simulink model "robot_model"  (R2025a)
settings: Solver=ode45  StartTime=0  StopTime=17  FixedStep=0.001  MaxStep=0.001  RelTol=1e-3
values from neighbouring files (symbols this model uses):
  K = table_of_controller_parameters(i).K    [plot_mesh_K.m]    (also in run_lqr_controller_optimization.m = table_of_controller_parameters(idx).K; run_the_robot_model.m = table_of_controller_parameters(idx).K)
  model_parameters = define_model_parameters()    [run_startup.m]    (also in startup.m)
libraries: simulink x6
settings Model: Creator=brzan  LastModifiedBy=brzan

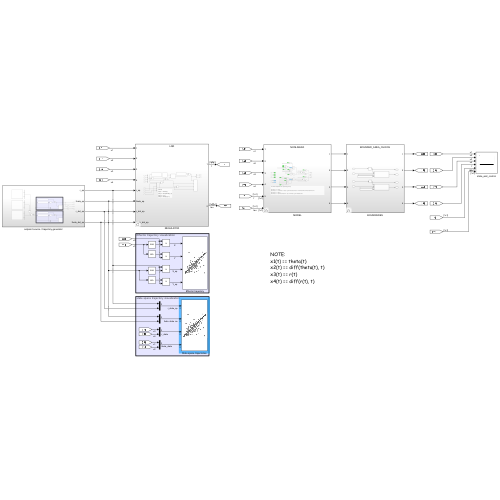
[thumbnail: Simulink's stored preview of the top-level diagram]
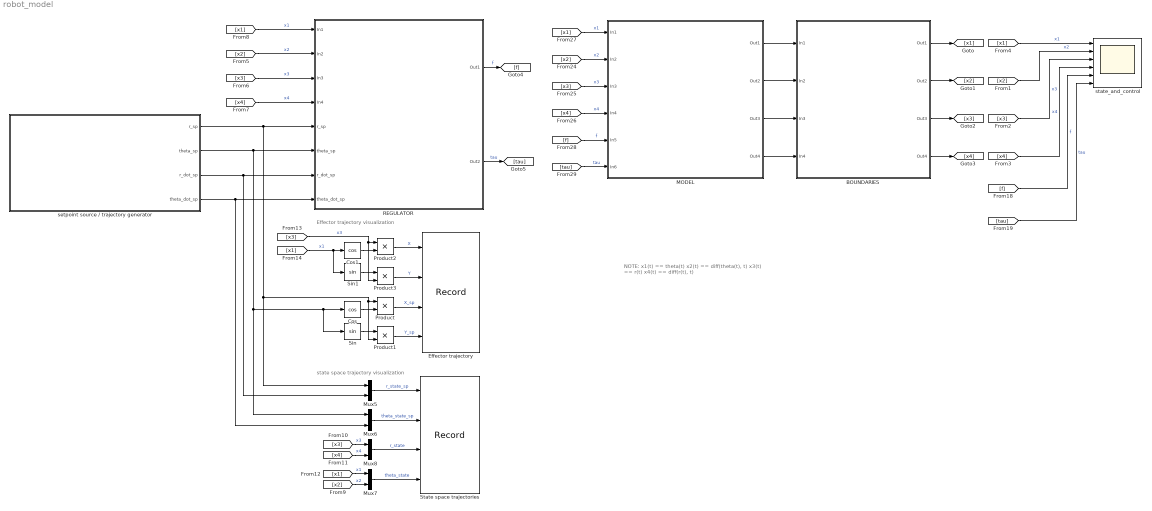
== system robot_model ==
  note: Effector trajectory visualization
  note: NOTE:
      | x1(t) == theta(t)
      | x2(t) == diff(theta(t), t)
      | x3(t) == r(t)
      | x4(t) == diff(r(t), t)
  note: state space trajectory visualization
  BOUNDARIES : Subsystem  Variant=on
  Cos : Trigonometry  Operator=cos
  Cos1 : Trigonometry  Operator=cos
  Effector trajectory : Record  NumPorts=4.0  FileSettingsInternal="{\"entries\":[{\"content\":{\"excelSettings\":{\"content\":{},\"type\":\"Streamout.ExcelSettings\"},\"parquetSettings\":{\"content\":{},\"type\":\"Streamout.ParquetSettings\"}},\"type\":\"Streamout.FileSettingStorage\",\"uuid\":\"\"}],\"packageUris\":[\"http:\\/\\/schema.mathworks.com\\/mf0\\/streamout_blocks\\/R2020a\"],\"version\":\"1.0\"}"  FrameSettings=[0, 0, 0, 0]  Layout=[1 2]  SignalsInternal="{\"entries\":[{\"content\":{\"signals\":[{\"content\":{\"blockPath\":[],\"dimensions\":[1],\"domain\":\"\",\"lineColor\":\"#0072bd\",\"plots\":[ 1 ],\"port\":1,\"sid\":[\"\"],\"signalID\":1,\"signalName\":\"X\"},\"type\":\"RecordBlkView.Signal\",\"uuid\":\"\"},{\"content\":{\"blockPath\":[],\"dimensions\":[1],\"domain\":\"\",\"lineColor\":\"#139fff\",\"plots\":[ 1 ],\"port\":2,\"sid\":[\"\"],\"signalID\":2,\"signalName\":\"Y\"},\"type\":\"RecordBlkView.Signal\",\"uuid\":\"\"},{\"content\":{\"blockPath\":[],\"dimensions\":[1],\"domain\":\"\",\"lineColor\":\"#d95319\",\"lineWidth\":2,\"plots\":[ 1 ],\"port\":3,\"sid\":[\"\"],\"signalID\":3,\"signalName\":\"X_sp\"},\"type\":\"RecordBlkView.Signal\",\"uuid\":\"\"},{\"content\":{\"blockPath\":[],\"dimensions\":[1],\"domain\":\"\",\"lineColor\":\"#ff6929\",\"lineWidth\":2,\"plots\":[ 1 ],\"port\":4,\"sid\":[\"\"],\"signalID\":4,\"signalName\":\"Y_sp\"},\"type\":\"RecordBlkView.Signal\",\"uuid\":\"\"}]},\"type\":\"RecordBlkView.InputSignals\",\"uuid\":\"\"}],\"packageUris\":[\"http:\\/\\/schema.mathworks.com\\/mf0\\/streamout_blocks\\/R2020a\"],\"version\":\"1.0\"}"  VisualizationBindings="{\"xyplotplugin\":{\"info\":[{\"series\":[{\"bindingParametersList\":[{\"parameter\":\"X-Axis\",\"signalID\":1,\"signalName\":\"X\"},{\"parameter\":\"Y-Axis\",\"signalID\":2,\"signalName\":\"Y\"}],\"seriesID\":0},{\"bindingParametersList\":[{\"parameter\":\"X-Axis\",\"signalID\":3,\"signalName\":\"X_sp\"},{\"parameter\":\"Y-Axis\",\"signalID\":4,\"signalName\":\"Y_sp\"}],\"seriesID\":1}],\"subplotID\":1}]}}"  CompatibilityTag=XY
  MODEL : Subsystem  Variant=on
  Mux{5..8} (4 alike) : Mux  Inputs=2
  Product{,1..3} (4 alike) : Product
  REGULATOR : Subsystem  Variant=on
  Sin : Trigonometry
  Sin1 : Trigonometry
  State space trajectories : Record  NumPorts=4.0  FileSettingsInternal="{\"entries\":[{\"content\":{\"excelSettings\":{\"content\":{},\"type\":\"Streamout.ExcelSettings\"},\"parquetSettings\":{\"content\":{},\"type\":\"Streamout.ParquetSettings\"}},\"type\":\"Streamout.FileSettingStorage\",\"uuid\":\"\"}],\"packageUris\":[\"http:\\/\\/schema.mathworks.com\\/mf0\\/streamout_blocks\\/R2020a\"],\"version\":\"1.0\"}"  FrameSettings=[0, 0, 0, 0]  Layout=[2 2]  SignalsInternal="{\"entries\":[{\"content\":{\"signals\":[{\"content\":{\"blockPath\":[],\"dimensions\":[2],\"domain\":\"\",\"hasChildren\":true,\"lineColor\":\"#ff6929\",\"lineWidth\":2,\"port\":1,\"sid\":[\"\"],\"signalID\":1,\"signalName\":\"r_state_sp\"},\"type\":\"RecordBlkView.Signal\",\"uuid\":\"\"},{\"content\":{\"blockPath\":[],\"channel\":[1],\"dimensions\":[2],\"domain\":\"\",\"lineColor\":\"#ff13a6\",\"lineWidth\":2,\"parentID\":1,\"plots\":[ 1, 9 ],\"port\":1,\"sid\":[\"\"],\"signalID\":2,\"signalName\":\"r_state_sp\"},\"type\":\"RecordBlkView.Signal\",\"uuid\":\"\"},{\"content\":{\"blockPath\":[],\"dimensions\":[2],\"domain\":\"\",\"hasChildren\":true,\"lineColor\":\"#64d413\",\"lineWidth\":2,\"port\":2,\"sid\":[\"\"],\"signalID\":3,\"signalName\":\"theta_state_sp\"},\"type\":\"RecordBlkView.Signal\",\"uuid\":\"\"},{\"content\":{\"blockPath\":[],\"channel\":[1],\"dimensions\":[2],\"domain\":\"\",\"lineColor\":\"#22b573\",\"lineWidth\":2,\"parentID\":3,\"plots\":[ 2, 10, 23 ],\"port\":2,\"sid\":[\"\"],\"signalID\":4,\"signalName\":\"theta_state_sp\"},\"type\":\"RecordBlkView.Signal\",\"uuid\":\"\"},{\"content\":{\"blockPath\":[],\"dimensions\":[2],\"domain\":\"\",\"hasChildren\":true,\"lineColor\":\"#fe330a\",\"lineWidth\":2,\"port\":3,\"sid\":[\"\"],\"signalID\":5,\"signalName\":\"r_state\"},\"type\":\"RecordBlkView.Signal\",\"uuid\":\"\"},{\"content\":{\"blockPath\":[],\"channel\":[1],\"dimensions\":[2],\"domain\":\"\",\"lineColor\":\"#d95319\",\"lineWidth\":2,\"parentID\":5,\"plots\":[ 1, 3, 5, 9, 25 ],\"port\":3,\"sid\":[\"\"],\"signalID\":6,\"signalName\":\"r_state\"},\"type\":\"RecordBlkView.Signal\",\"uuid\":\"\"},{\"content\":{\"blockPath\":[],\"dimensions\":[2],\"domain\":\"\",\"hasChildren\":true,\"lineColor\":\"#0072bd\",\"lineWidth\":2,\"port\":4,\"sid\":[\"\"],\"signalID\":7,\"signalName\":\"theta_state\"},\"type\":\"RecordBlkView.Signal\",\"uuid\":\"\"},{\"content\":{\"blockPath\":[],\"channel\":[1],\"dimensions\":[2],\"domain\":\"\",\"lineColor\":\"#7e2f8e\",\"lineWidth\":2,\"parentID\":7,\"plots\":[ 2, 10, 26, 51 ],\"port\":4,\"sid\":[\"\"],\"signalID\":8,\"signalName\":\"theta_state\"},\"type\":\"RecordBlkView.Signal\",\"uuid\":\"\"},{\"content\":{\"blockPath\":[],\"channel\":[2],\"dimensions\":[2],\"domain\":\"\",\"lineColor\":\"#fe330a\",\"lineWidth\":2,\"parentID\":1,\"plots\":[ 1, 9, 15, 48 ],\"port\":1,\"sid\":[\"\"],\"signalID\":9,\"signalName\":\"r_state_sp\"},\"type\":\"RecordBlkView.Signal\",\"uuid\":\"\"},{\"content\":{\"blockPath\":[],\"channel\":[2],\"dimensions\":[2],\"domain\":\"\",\"lineColor\":\"#22b573\",\"lineWidth\":2,\"parentID\":3,\"plots\":[ 2, 10, 58, 59 ],\"port\":2,\"sid\":[\"\"],\"signalID\":10,\"signalName\":\"theta_state_sp\"},\"type\":\"RecordBlkView.Signal\",\"uuid\":\"\"},{\"content\":{\"blockPath\":[],\"channel\":[2],\"dimensions\":[2],\"domain\":\"\",\"lineColor\":\"#0072bd\",\"lineWidth\":2,\"parentID\":5,\"plots\":[ 1, 9, 41 ],\"port\":3,\"sid\":[\"\"],\"signalID\":11,\"signalName\":\"r_state\"},\"type\":\"RecordBlkView.Signal\",\"uuid\":\"\"},{\"content\":{\"blockPath\":[],\"channel\":[2],\"dimensions\":[2],\"domain\":\"\",\"lineColor\":\"#d95319\",\"lineWidth\":2,\"parentID\":7,\"plots\":[ 2, 10, 45 ],\"port\":4,\"sid\":[\"\"],\"signalID\":12,\"signalName\":\"theta_state\"},\"type\":\"RecordBlkView.Signal\",\"uuid\":\"\"}]},\"type\":\"RecordBlkView.InputSignals\",\"uuid\":\"\"}],\"packageUris\":[\"http:\\/\\/schema.mathworks.com\\/mf0\\/streamout_blocks\\/R2020a\"],\"version\":\"1.0\"}"  VisualizationBindings="{\"sparklinesplugin\":{\"info\":[{\"bindingParametersList\":[],\"subplotID\":9},{\"bindingParametersList\":[],\"subplotID\":10}]},\"xyplotplugin\":{\"info\":[{\"series\":[{\"bindingParametersList\":[{\"parameter\":\"X-Axis\",\"signalID\":2,\"signalName\":\"r_state_sp(1)\"},{\"parameter\":\"Y-Axis\",\"signalID\":9,\"signalName\":\"r_state_sp(2)\"}],\"seriesID\":0},{\"bindingParametersList\":[{\"parameter\":\"X-Axis\",\"signalID\":6,\"signalName\":\"r_state(1)\"},{\"parameter\":\"Y-Axis\",\"signalID\":11,\"signalName\":\"r_state(2)\"}],\"seriesID\":1}],\"subplotID\":1},{\"series\":[{\"bindingParametersList\":[{\"parameter\":\"X-Axis\",\"signalID\":4,\"signalName\":\"theta_state_sp(1)\"},{\"parameter\":\"Y-Axis\",\"signalID\":10,\"signalName\":\"theta_state_sp(2)\"}],\"seriesID\":2},{\"bindingParametersList\":[{\"parameter\":\"X-Axis\",\"signalID\":8,\"signalName\":\"theta_state(1)\"},{\"parameter\":\"Y-Axis\",\"signalID\":12,\"signalName\":\"theta_state(2)\"}],\"seriesID\":3}],\"subplotID\":2}]}}"  CompatibilityTag=XY
  setpoint source / trajectory generator : Subsystem
  state_and_control : Scope  NumInputPorts=6
      settings: ActiveDisplayYMinimum=2.4867230453181195  ActiveDisplayYMaximum=2.7484021064636068  DataLoggingVariableName=state_and_control
  wires:
  [x4] -> state_and_control/4  "x4"
  [x3] -> state_and_control/3  "x3"
  [x2] -> state_and_control/2  "x2"
  [x1] -> state_and_control/1  "x1"
  [f] -> state_and_control/5  "f"
  [tau] -> state_and_control/6  "tau"
  MODEL/1(Out1) -> BOUNDARIES/1(In1)
  MODEL/2(Out2) -> BOUNDARIES/2(In2)
  MODEL/3(Out3) -> BOUNDARIES/3(In3)
  MODEL/4(Out4) -> BOUNDARIES/4(In4)
  BOUNDARIES/1(Out1) -> [x1]
  BOUNDARIES/2(Out2) -> [x2]
  BOUNDARIES/3(Out3) -> [x3]
  BOUNDARIES/4(Out4) -> [x4]
  [x4] -> MODEL/4(In4)  "x4"
  [x3] -> MODEL/3(In3)  "x3"
  [x2] -> MODEL/2(In2)  "x2"
  [x1] -> MODEL/1(In1)  "x1"
  [f] -> MODEL/5(In5)  "f"
  [tau] -> MODEL/6(In6)  "tau"
  REGULATOR/2(Out2) -> [tau]  "tau"
  REGULATOR/1(Out1) -> [f]  "f"
  [x1] -> REGULATOR/1(In1)  "x1"
  [x2] -> REGULATOR/2(In2)  "x2"
  [x3] -> REGULATOR/3(In3)  "x3"
  [x4] -> REGULATOR/4(In4)  "x4"
  Cos/1 -> Product/2
  Sin/1 -> Product1/1
  Product/1 -> Effector trajectory/3  "X_sp"
  Product1/1 -> Effector trajectory/4  "Y_sp"
  Mux5/1 -> State space trajectories/1  "r_state_sp"
  Mux6/1 -> State space trajectories/2  "theta_state_sp"
  Mux8/1 -> State space trajectories/3  "r_state"
  Mux7/1 -> State space trajectories/4  "theta_state"
  [x1] -> Mux7/1  "x1"
  [x2] -> Mux7/2  "x2"
  [x4] -> Mux8/2  "x4"
  [x3] -> Mux8/1  "x3"
  [x1] -> Sin1/1, Cos1/1  "x1"
  [x3] -> Product3/2, Product2/1  "x3"
  Sin1/1 -> Product3/1
  Cos1/1 -> Product2/2
  Product3/1 -> Effector trajectory/2  "Y"
  Product2/1 -> Effector trajectory/1  "X"
  setpoint source / trajectory generator/2(theta_sp) -> Mux6/1, Cos/1, Sin/1, REGULATOR/6(theta_sp)
  setpoint source / trajectory generator/1(r_sp) -> Mux5/1, Product1/2, Product/1, REGULATOR/5(r_sp)
  setpoint source / trajectory generator/3(r_dot_sp) -> Mux5/2, REGULATOR/7(r_dot_sp)
  setpoint source / trajectory generator/4(theta_dot_sp) -> Mux6/2, REGULATOR/8(theta_dot_sp)

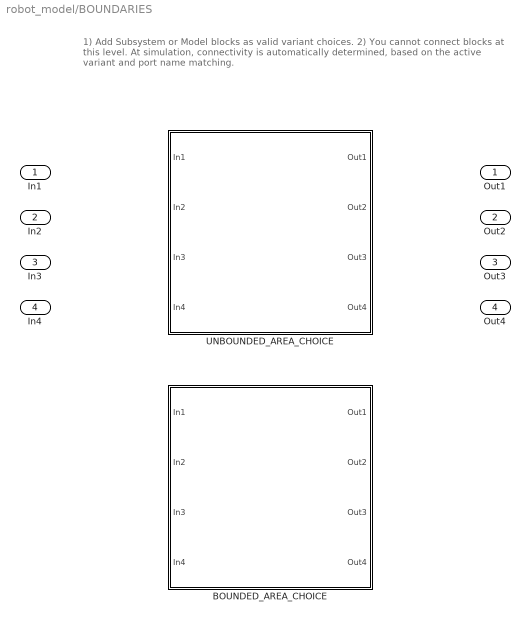
== system robot_model/BOUNDARIES ==
  note: 1) Add Subsystem or Model blocks as valid variant choices.
      | 2) You cannot connect blocks at this level. At simulation, connectivity is automatically
      | determined, based on the active variant and port name matching.
  In1 : Inport
  In2 : Inport  Port=2
  In3 : Inport  Port=3
  In4 : Inport  Port=4
  BOUNDED_AREA_CHOICE : Subsystem  VariantControl="BOUNDARY_CHOICE == \"BOUNDED\""
  UNBOUNDED_AREA_CHOICE : Subsystem  VariantControl="BOUNDARY_CHOICE == \"UNBOUNDED\""
  Out1 : Outport
  Out2 : Outport  Port=2
  Out3 : Outport  Port=3
  Out4 : Outport  Port=4

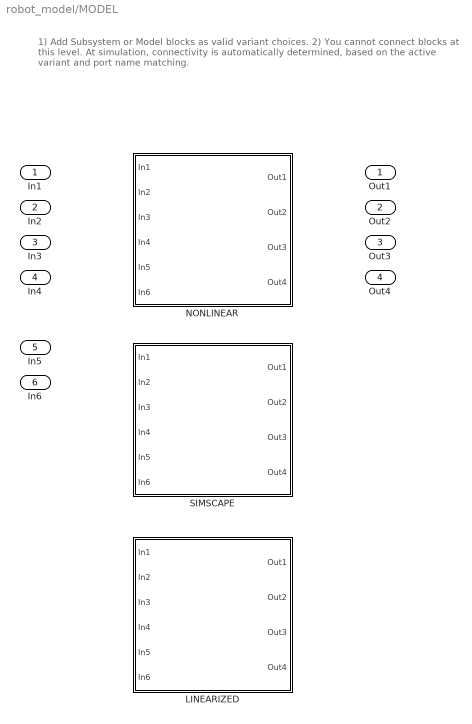
== system robot_model/MODEL ==
  note: 1) Add Subsystem or Model blocks as valid variant choices.
      | 2) You cannot connect blocks at this level. At simulation, connectivity is automatically
      | determined, based on the active variant and port name matching.
  In1 : Inport
  In2 : Inport  Port=2
  In3 : Inport  Port=3
  In4 : Inport  Port=4
  In5 : Inport  Port=5
  In6 : Inport  Port=6
  LINEARIZED : Subsystem  VariantControl="MODEL_CHOICE == \"LINEARIZED\""
  NONLINEAR : Subsystem  VariantControl="MODEL_CHOICE == \"NONLINEAR\""
  SIMSCAPE : Subsystem  VariantControl="MODEL_CHOICE == \"SIMSCAPE\""
  Out1 : Outport
  Out2 : Outport  Port=2
  Out3 : Outport  Port=3
  Out4 : Outport  Port=4

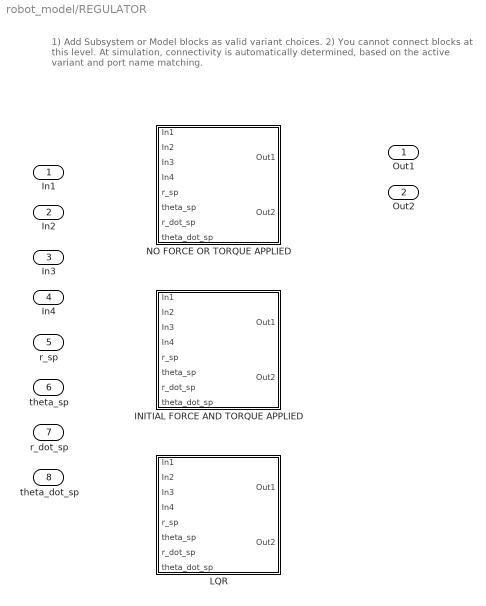
== system robot_model/REGULATOR ==
  note: 1) Add Subsystem or Model blocks as valid variant choices.
      | 2) You cannot connect blocks at this level. At simulation, connectivity is automatically
      | determined, based on the active variant and port name matching.
  In1 : Inport
  In2 : Inport  Port=2
  In3 : Inport  Port=3
  In4 : Inport  Port=4
  r_sp : Inport  Port=5
  theta_sp : Inport  Port=6
  r_dot_sp : Inport  Port=7
  theta_dot_sp : Inport  Port=8
  INITIAL FORCE AND TORQUE APPLIED : Subsystem  VariantControl="REGULATOR_CHOICE == \"INITIAL_FORCE_AND_TORQUE_APPLIED\""
  LQR : Subsystem  VariantControl="REGULATOR_CHOICE == \"LQR\""
  NO FORCE OR TORQUE APPLIED : Subsystem  VariantControl="REGULATOR_CHOICE == \"NO_FORCE_AND_TORQUE_APPLIED\""
  Out1 : Outport
  Out2 : Outport  Port=2

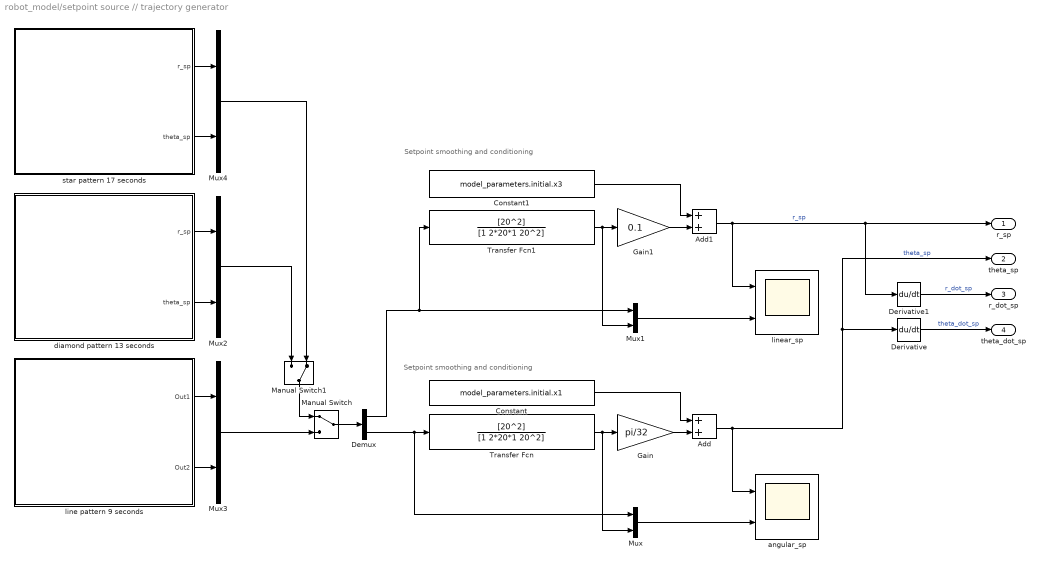
== system robot_model/setpoint source // trajectory generator ==
  note: Setpoint smoothing and conditioning
  note: Setpoint smoothing and conditioning
  Add : Sum
  Add1 : Sum
  Constant : Constant  Value=model_parameters.initial.x1
  Constant1 : Constant  Value=model_parameters.initial.x3
  Demux : Demux  Outputs=2
  Derivative : Derivative
  Derivative1 : Derivative
  Gain : Gain  Gain=pi/32
  Gain1 : Gain  Gain=0.1
  Manual Switch : ManualSwitch
  Manual Switch1 : ManualSwitch  CurrentSetting=0
  Mux{,1..4} (5 alike) : Mux  Inputs=2
  Transfer Fcn : TransferFcn  Numerator=[20^2]  Denominator=[1 2*20*1 20^2]
  Transfer Fcn1 : TransferFcn  Numerator=[20^2]  Denominator=[1 2*20*1 20^2]
  angular_sp : Scope  NumInputPorts=2
      settings: ActiveDisplayYMinimum=-1  ActiveDisplayYMaximum=1  DataLoggingVariableName=angular_sp
  diamond pattern 13 seconds : Subsystem
  line pattern 9 seconds : Subsystem
  linear_sp : Scope  NumInputPorts=2
      settings: ActiveDisplayYMinimum=-1  ActiveDisplayYMaximum=1  DataLoggingVariableName=linear_sp
  star pattern 17 seconds : Subsystem
  r_sp : Outport
  theta_sp : Outport  Port=2
  r_dot_sp : Outport  Port=3
  theta_dot_sp : Outport  Port=4
  wires:
  Mux4/1 -> Manual Switch1/2
  Add1/1 -> linear_sp/1, r_sp/1, Derivative1/1  "r_sp"
  diamond pattern 13 seconds/2(theta_sp) -> Mux2/2
  Transfer Fcn/1 -> Mux/2, Gain/1
  Derivative1/1 -> r_dot_sp/1  "r_dot_sp"
  Gain1/1 -> Add1/2
  Add/1 -> angular_sp/1, theta_sp/1, Derivative/1  "theta_sp"
  star pattern 17 seconds/2(theta_sp) -> Mux4/2
  Mux2/1 -> Manual Switch1/1
  Mux1/1 -> linear_sp/2
  Constant/1 -> Add/1
  Demux/2 -> Mux/1, Transfer Fcn/1
  Manual Switch/1 -> Demux/1
  Transfer Fcn1/1 -> Mux1/2, Gain1/1
  diamond pattern 13 seconds/1(r_sp) -> Mux2/1
  Constant1/1 -> Add1/1
  line pattern 9 seconds/2(Out2) -> Mux3/2
  Mux3/1 -> Manual Switch/2
  Demux/1 -> Mux1/1, Transfer Fcn1/1
  star pattern 17 seconds/1(r_sp) -> Mux4/1
  Derivative/1 -> theta_dot_sp/1  "theta_dot_sp"
  Gain/1 -> Add/2
  line pattern 9 seconds/1(Out1) -> Mux3/1
  Mux/1 -> angular_sp/2
  Manual Switch1/1 -> Manual Switch/1

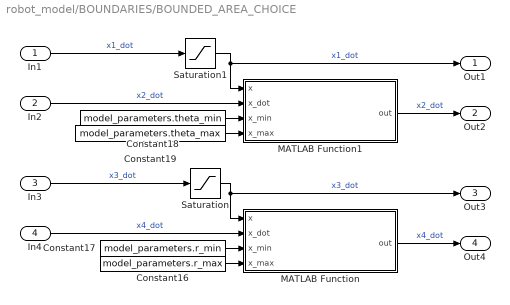
== system robot_model/BOUNDARIES/BOUNDED_AREA_CHOICE ==
  In1 : Inport
  In2 : Inport  Port=2
  In3 : Inport  Port=3
  In4 : Inport  Port=4
  Constant16 : Constant  Value=model_parameters.r_max
  Constant17 : Constant  Value=model_parameters.r_min
  Constant18 : Constant  Value=model_parameters.theta_min
  Constant19 : Constant  Value=model_parameters.theta_max
  MATLAB Function : MATLAB Function  TreatAsAtomicUnit=on
  MATLAB Function1 : MATLAB Function  TreatAsAtomicUnit=on
  Saturation : Saturate  UpperLimit=model_parameters.r_max  LowerLimit=model_parameters.r_min
  Saturation1 : Saturate  UpperLimit=model_parameters.theta_max  LowerLimit=model_parameters.theta_min
  Out1 : Outport
  Out2 : Outport  Port=2
  Out3 : Outport  Port=3
  Out4 : Outport  Port=4
  wires:
  In3/1 -> Saturation/1  "x3_dot"
  Constant18/1 -> MATLAB Function1/3(x_min)
  In1/1 -> Saturation1/1  "x1_dot"
  Saturation1/1 -> Out1/1, MATLAB Function1/1(x)  "x1_dot"
  Saturation/1 -> Out3/1, MATLAB Function/1(x)  "x3_dot"
  Constant17/1 -> MATLAB Function/3(x_min)
  Constant16/1 -> MATLAB Function/4(x_max)
  Constant19/1 -> MATLAB Function1/4(x_max)
  MATLAB Function1/1(out) -> Out2/1  "x2_dot"
  In2/1 -> MATLAB Function1/2(x_dot)  "x2_dot"
  In4/1 -> MATLAB Function/2(x_dot)  "x4_dot"
  MATLAB Function/1(out) -> Out4/1  "x4_dot"

== system robot_model/BOUNDARIES/UNBOUNDED_AREA_CHOICE ==
  In1 : Inport
  In2 : Inport  Port=2
  In3 : Inport  Port=3
  In4 : Inport  Port=4
  Out1 : Outport
  Out2 : Outport  Port=2
  Out3 : Outport  Port=3
  Out4 : Outport  Port=4
  wires:
  In1/1 -> Out1/1
  In2/1 -> Out2/1
  In3/1 -> Out3/1
  In4/1 -> Out4/1

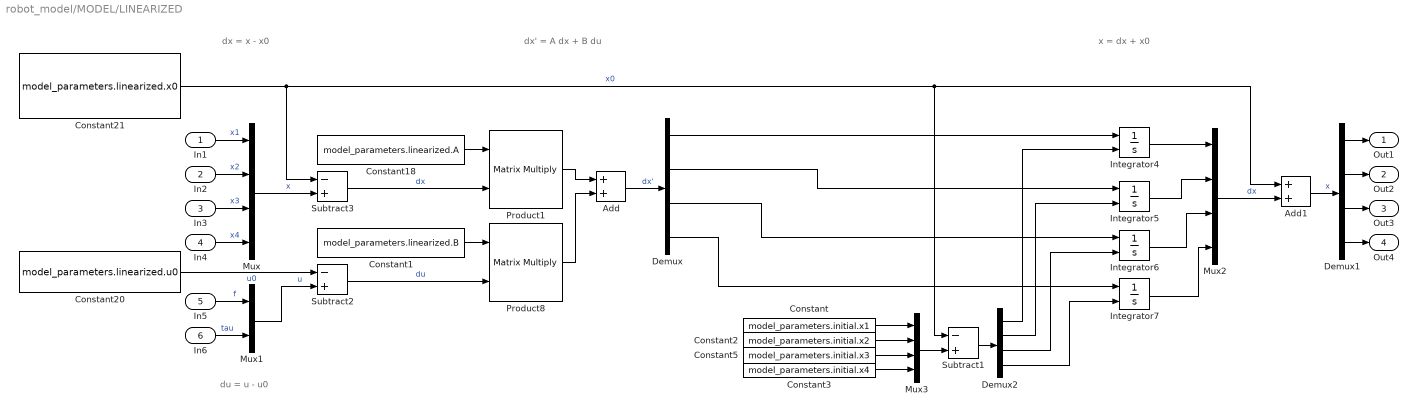
== system robot_model/MODEL/LINEARIZED ==
  note: du = u - u0
  note: dx = x - x0
  note: x = dx + x0
  note: dx' = A dx + B du
  In1 : Inport
  In2 : Inport  Port=2
  In3 : Inport  Port=3
  In4 : Inport  Port=4
  In5 : Inport  Port=5
  In6 : Inport  Port=6
  Add : Sum
  Add1 : Sum
  Constant : Constant  Value=model_parameters.initial.x1
  Constant1 : Constant  Value=model_parameters.linearized.B  VectorParams1D=off
  Constant18 : Constant  Value=model_parameters.linearized.A  VectorParams1D=off
  Constant2 : Constant  Value=model_parameters.initial.x2
  Constant20 : Constant  Value=model_parameters.linearized.u0  VectorParams1D=off
  Constant21 : Constant  Value=model_parameters.linearized.x0  VectorParams1D=off
  Constant3 : Constant  Value=model_parameters.initial.x4
  Constant5 : Constant  Value=model_parameters.initial.x3
  Demux : Demux
  Demux1 : Demux
  Demux2 : Demux
  Integrator{4..7} (4 alike) : Integrator  InitialConditionSource=external
  Mux : Mux
  Mux1 : Mux  Inputs=2
  Mux2 : Mux
  Mux3 : Mux
  Product1 : Product  Multiplication=Matrix(*)
  Product8 : Product  Multiplication=Matrix(*)
  Subtract1 : Sum  Inputs=-+
  Subtract2 : Sum  Inputs=-+
  Subtract3 : Sum  Inputs=-+
  Out1 : Outport
  Out2 : Outport  Port=2
  Out3 : Outport  Port=3
  Out4 : Outport  Port=4
  wires:
  In1/1 -> Mux/1  "x1"
  Integrator7/1 -> Mux2/4
  Demux/3 -> Integrator6/1
  Integrator6/1 -> Mux2/3
  Demux/2 -> Integrator5/1
  Demux2/3 -> Integrator6/2
  Product1/1 -> Add/1
  Integrator5/1 -> Mux2/2
  Demux2/1 -> Integrator4/2
  Mux1/1 -> Subtract2/2  "u"
  Demux1/3 -> Out3/1
  Mux2/1 -> Add1/2  "dx"
  Constant1/1 -> Product8/1
  Constant18/1 -> Product1/1
  Constant20/1 -> Subtract2/1  "u0"
  Demux/4 -> Integrator7/1
  Demux1/4 -> Out4/1
  Demux2/4 -> Integrator7/2
  Mux/1 -> Subtract3/2  "x"
  Constant21/1 -> Subtract1/1, Add1/1, Subtract3/1  "x0"
  Demux1/1 -> Out1/1
  Product8/1 -> Add/2
  Demux1/2 -> Out2/1
  Integrator4/1 -> Mux2/1
  Add1/1 -> Demux1/1  "x"
  Subtract2/1 -> Product8/2  "du"
  Add/1 -> Demux/1  "dx'"
  Demux2/2 -> Integrator5/2
  Subtract3/1 -> Product1/2  "dx"
  Demux/1 -> Integrator4/1
  In2/1 -> Mux/2  "x2"
  In3/1 -> Mux/3  "x3"
  In4/1 -> Mux/4  "x4"
  In5/1 -> Mux1/1  "f"
  In6/1 -> Mux1/2  "tau"
  Constant2/1 -> Mux3/2
  Constant5/1 -> Mux3/3
  Constant/1 -> Mux3/1
  Constant3/1 -> Mux3/4
  Mux3/1 -> Subtract1/2
  Subtract1/1 -> Demux2/1

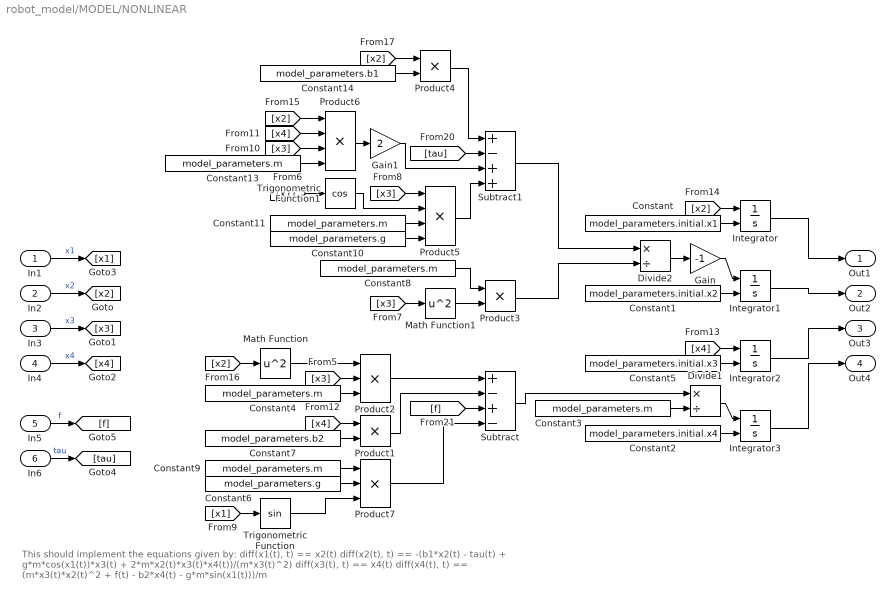
== system robot_model/MODEL/NONLINEAR ==
  note: This should implement the equations given by:
      |
      | diff(x1(t), t) == x2(t)
      | diff(x2(t), t) == -(b1*x2(t) - tau(t) + g*m*cos(x1(t))*x3(t) + 2*m*x2(t)*x3(t)*x4(t))/(m*x3(t)^2)
      | diff(x3(t), t) == x4(t)
      | diff(x4(t), t) == (m*x3(t)*x2(t)^2 + f(t) - b2*x4(t) - g*m*sin(x1(t)))/m
  In1 : Inport
  In2 : Inport  Port=2
  In3 : Inport  Port=3
  In4 : Inport  Port=4
  In5 : Inport  Port=5
  In6 : Inport  Port=6
  Constant : Constant  Value=model_parameters.initial.x1
  Constant1 : Constant  Value=model_parameters.initial.x2
  Constant10 : Constant  Value=model_parameters.g
  Constant{3..4,8..9,11,13} (6 alike) : Constant  Value=model_parameters.m
  Constant14 : Constant  Value=model_parameters.b1
  Constant2 : Constant  Value=model_parameters.initial.x4
  Constant5 : Constant  Value=model_parameters.initial.x3
  Constant6 : Constant  Value=model_parameters.g
  Constant7 : Constant  Value=model_parameters.b2
  Divide1 : Product  Inputs=*/
  Divide2 : Product  Inputs=*/
  Gain : Gain  Gain=-1
  Gain1 : Gain  Gain=2
  Integrator{,1..3} (4 alike) : Integrator  InitialConditionSource=external
  Math Function : Math  Operator=square
  Math Function1 : Math  Operator=square
  Product1 : Product
  Product2 : Product  Inputs=3
  Product3 : Product
  Product4 : Product
  Product5 : Product  Inputs=4
  Product6 : Product  Inputs=4
  Product7 : Product  Inputs=3
  Subtract : Sum  Inputs=+-+-
  Subtract1 : Sum  Inputs=+-++
  Trigonometric Function : Trigonometry
  Trigonometric Function1 : Trigonometry  Operator=cos
  Out1 : Outport
  Out2 : Outport  Port=2
  Out3 : Outport  Port=3
  Out4 : Outport  Port=4
  wires:
  Constant6/1 -> Product7/2
  Product7/1 -> Subtract/4
  Subtract1/1 -> Divide2/1
  Product2/1 -> Subtract/1
  Constant13/1 -> Product6/4
  [f] -> Subtract/3
  Constant4/1 -> Product2/3
  [x3] -> Product2/2
  [tau] -> Subtract1/2
  Constant14/1 -> Product4/2
  Product1/1 -> Subtract/2
  Constant8/1 -> Product3/1
  Math Function1/1 -> Product3/2
  Divide2/1 -> Gain/1
  Subtract/1 -> Divide1/1
  Product3/1 -> Divide2/2
  Gain1/1 -> Subtract1/3
  [x2] -> Product4/1
  Constant9/1 -> Product7/1
  Constant11/1 -> Product5/3
  [x1] -> Trigonometric Function/1
  Product5/1 -> Subtract1/4
  Product4/1 -> Subtract1/1
  Math Function/1 -> Product2/1
  [x4] -> Product6/2
  Constant3/1 -> Divide1/2
  Trigonometric Function/1 -> Product7/3
  [x4] -> Product1/1
  Product6/1 -> Gain1/1
  [x2] -> Math Function/1
  [x3] -> Product5/1
  Constant7/1 -> Product1/2
  [x2] -> Product6/1
  Trigonometric Function1/1 -> Product5/2
  [x1] -> Trigonometric Function1/1
  Constant10/1 -> Product5/4
  [x3] -> Product6/3
  In2/1 -> [x2]  "x2"
  In3/1 -> [x3]  "x3"
  In4/1 -> [x4]  "x4"
  In1/1 -> [x1]  "x1"
  In6/1 -> [tau]  "tau"
  In5/1 -> [f]  "f"
  Constant/1 -> Integrator/2
  Constant5/1 -> Integrator2/2
  Gain/1 -> Integrator1/1
  [x4] -> Integrator2/1
  [x2] -> Integrator/1
  Divide1/1 -> Integrator3/1
  Constant1/1 -> Integrator1/2
  Constant2/1 -> Integrator3/2
  Integrator/1 -> Out1/1
  Integrator1/1 -> Out2/1
  Integrator2/1 -> Out3/1
  Integrator3/1 -> Out4/1
  [x3] -> Math Function1/1

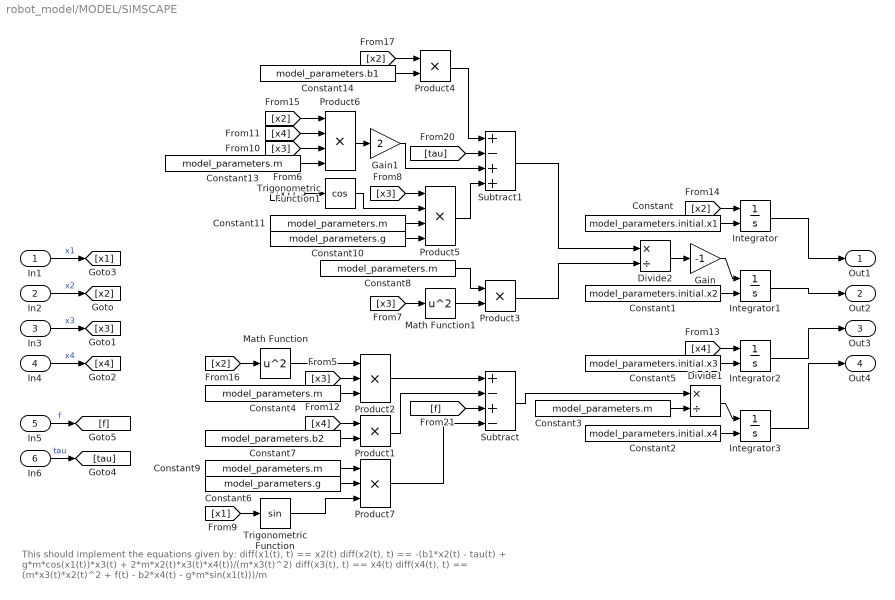
== system robot_model/MODEL/SIMSCAPE ==
  note: This should implement the equations given by:
      |
      | diff(x1(t), t) == x2(t)
      | diff(x2(t), t) == -(b1*x2(t) - tau(t) + g*m*cos(x1(t))*x3(t) + 2*m*x2(t)*x3(t)*x4(t))/(m*x3(t)^2)
      | diff(x3(t), t) == x4(t)
      | diff(x4(t), t) == (m*x3(t)*x2(t)^2 + f(t) - b2*x4(t) - g*m*sin(x1(t)))/m
  In1 : Inport
  In2 : Inport  Port=2
  In3 : Inport  Port=3
  In4 : Inport  Port=4
  In5 : Inport  Port=5
  In6 : Inport  Port=6
  Constant : Constant  Value=model_parameters.initial.x1
  Constant1 : Constant  Value=model_parameters.initial.x2
  Constant10 : Constant  Value=model_parameters.g
  Constant{3..4,8..9,11,13} (6 alike) : Constant  Value=model_parameters.m
  Constant14 : Constant  Value=model_parameters.b1
  Constant2 : Constant  Value=model_parameters.initial.x4
  Constant5 : Constant  Value=model_parameters.initial.x3
  Constant6 : Constant  Value=model_parameters.g
  Constant7 : Constant  Value=model_parameters.b2
  Divide1 : Product  Inputs=*/
  Divide2 : Product  Inputs=*/
  Gain : Gain  Gain=-1
  Gain1 : Gain  Gain=2
  Integrator{,1..3} (4 alike) : Integrator  InitialConditionSource=external
  Math Function : Math  Operator=square
  Math Function1 : Math  Operator=square
  Product1 : Product
  Product2 : Product  Inputs=3
  Product3 : Product
  Product4 : Product
  Product5 : Product  Inputs=4
  Product6 : Product  Inputs=4
  Product7 : Product  Inputs=3
  Subtract : Sum  Inputs=+-+-
  Subtract1 : Sum  Inputs=+-++
  Trigonometric Function : Trigonometry
  Trigonometric Function1 : Trigonometry  Operator=cos
  Out1 : Outport
  Out2 : Outport  Port=2
  Out3 : Outport  Port=3
  Out4 : Outport  Port=4
  wires:
  Constant6/1 -> Product7/2
  Product7/1 -> Subtract/4
  Subtract1/1 -> Divide2/1
  Product2/1 -> Subtract/1
  Constant13/1 -> Product6/4
  [f] -> Subtract/3
  Constant4/1 -> Product2/3
  [x3] -> Product2/2
  [tau] -> Subtract1/2
  Constant14/1 -> Product4/2
  Product1/1 -> Subtract/2
  Constant8/1 -> Product3/1
  Math Function1/1 -> Product3/2
  Divide2/1 -> Gain/1
  Subtract/1 -> Divide1/1
  Product3/1 -> Divide2/2
  Gain1/1 -> Subtract1/3
  [x2] -> Product4/1
  Constant9/1 -> Product7/1
  Constant11/1 -> Product5/3
  [x1] -> Trigonometric Function/1
  Product5/1 -> Subtract1/4
  Product4/1 -> Subtract1/1
  Math Function/1 -> Product2/1
  [x4] -> Product6/2
  Constant3/1 -> Divide1/2
  Trigonometric Function/1 -> Product7/3
  [x4] -> Product1/1
  Product6/1 -> Gain1/1
  [x2] -> Math Function/1
  [x3] -> Product5/1
  Constant7/1 -> Product1/2
  [x2] -> Product6/1
  Trigonometric Function1/1 -> Product5/2
  [x1] -> Trigonometric Function1/1
  Constant10/1 -> Product5/4
  [x3] -> Product6/3
  In2/1 -> [x2]  "x2"
  In3/1 -> [x3]  "x3"
  In4/1 -> [x4]  "x4"
  In1/1 -> [x1]  "x1"
  In6/1 -> [tau]  "tau"
  In5/1 -> [f]  "f"
  Constant/1 -> Integrator/2
  Constant5/1 -> Integrator2/2
  Gain/1 -> Integrator1/1
  [x4] -> Integrator2/1
  [x2] -> Integrator/1
  Divide1/1 -> Integrator3/1
  Constant1/1 -> Integrator1/2
  Constant2/1 -> Integrator3/2
  Integrator/1 -> Out1/1
  Integrator1/1 -> Out2/1
  Integrator2/1 -> Out3/1
  Integrator3/1 -> Out4/1
  [x3] -> Math Function1/1

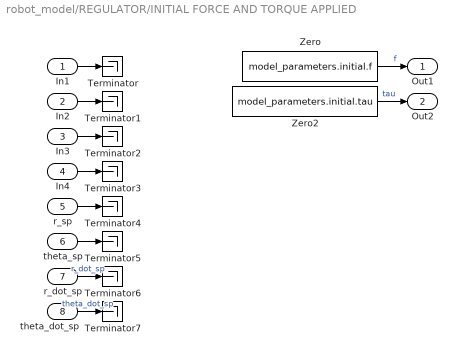
== system robot_model/REGULATOR/INITIAL FORCE AND TORQUE APPLIED ==
  In1 : Inport
  In2 : Inport  Port=2
  In3 : Inport  Port=3
  In4 : Inport  Port=4
  r_sp : Inport  Port=5
  theta_sp : Inport  Port=6
  r_dot_sp : Inport  Port=7
  theta_dot_sp : Inport  Port=8
  Terminator{,1..7} (8 alike) : Terminator
  Zero : Constant  Value=model_parameters.initial.f  OutDataTypeStr=Inherit: Inherit via back propagation
  Zero2 : Constant  Value=model_parameters.initial.tau  OutDataTypeStr=Inherit: Inherit via back propagation
  Out1 : Outport
  Out2 : Outport  Port=2
  wires:
  In1/1 -> Terminator/1
  In2/1 -> Terminator1/1
  In3/1 -> Terminator2/1
  In4/1 -> Terminator3/1
  Zero/1 -> Out1/1  "f"
  Zero2/1 -> Out2/1  "tau"
  r_sp/1 -> Terminator4/1
  theta_sp/1 -> Terminator5/1
  theta_dot_sp/1 -> Terminator7/1  "theta_dot_sp"
  r_dot_sp/1 -> Terminator6/1  "r_dot_sp"

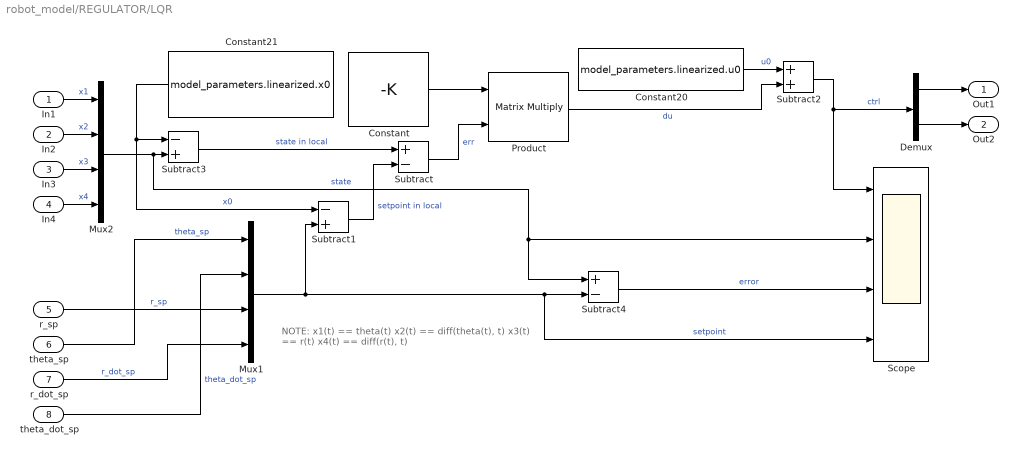
== system robot_model/REGULATOR/LQR ==
  note: NOTE:
      | x1(t) == theta(t)
      | x2(t) == diff(theta(t), t)
      | x3(t) == r(t)
      | x4(t) == diff(r(t), t)
  In1 : Inport
  In2 : Inport  Port=2
  In3 : Inport  Port=3
  In4 : Inport  Port=4
  r_sp : Inport  Port=5
  theta_sp : Inport  Port=6
  r_dot_sp : Inport  Port=7
  theta_dot_sp : Inport  Port=8
  Constant : Constant  Value=-K
  Constant20 : Constant  Value=model_parameters.linearized.u0  VectorParams1D=off
  Constant21 : Constant  Value=model_parameters.linearized.x0  VectorParams1D=off
  Demux : Demux  Outputs=2
  Mux1 : Mux
  Mux2 : Mux
  Product : Product  Multiplication=Matrix(*)
  Scope : Scope  NumInputPorts=4
      settings: ActiveDisplayYMinimum=-1  ActiveDisplayYMaximum=1
  Subtract : Sum  Inputs=+-
  Subtract1 : Sum  Inputs=-+
  Subtract2 : Sum
  Subtract3 : Sum  Inputs=-+
  Subtract4 : Sum  Inputs=+-
  Out1 : Outport
  Out2 : Outport  Port=2
  wires:
  Demux/1 -> Out1/1
  Demux/2 -> Out2/1
  Constant/1 -> Product/1
  r_sp/1 -> Mux1/3  "r_sp"
  theta_sp/1 -> Mux1/1  "theta_sp"
  theta_dot_sp/1 -> Mux1/2  "theta_dot_sp"
  r_dot_sp/1 -> Mux1/4  "r_dot_sp"
  Mux1/1 -> Scope/4, Subtract4/2, Subtract1/2  "setpoint"
  Subtract3/1 -> Subtract/1  "state in local"
  In1/1 -> Mux2/1  "x1"
  In2/1 -> Mux2/2  "x2"
  In3/1 -> Mux2/3  "x3"
  In4/1 -> Mux2/4  "x4"
  Subtract/1 -> Product/2  "err"
  Product/1 -> Subtract2/2  "du"
  Constant21/1 -> Subtract3/1, Subtract1/1  "x0"
  Mux2/1 -> Subtract4/1, Scope/2, Subtract3/2  "state"
  Constant20/1 -> Subtract2/1  "u0"
  Subtract2/1 -> Scope/1, Demux/1  "ctrl"
  Subtract1/1 -> Subtract/2  "setpoint in local"
  Subtract4/1 -> Scope/3  "error"

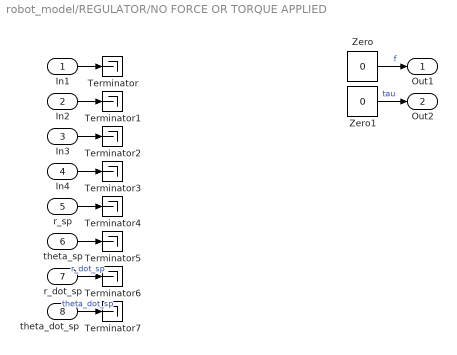
== system robot_model/REGULATOR/NO FORCE OR TORQUE APPLIED ==
  In1 : Inport
  In2 : Inport  Port=2
  In3 : Inport  Port=3
  In4 : Inport  Port=4
  r_sp : Inport  Port=5
  theta_sp : Inport  Port=6
  r_dot_sp : Inport  Port=7
  theta_dot_sp : Inport  Port=8
  Terminator{,1..7} (8 alike) : Terminator
  Zero : Constant  Value=0  OutDataTypeStr=Inherit: Inherit via back propagation
  Zero1 : Constant  Value=0  OutDataTypeStr=Inherit: Inherit via back propagation
  Out1 : Outport
  Out2 : Outport  Port=2
  wires:
  In1/1 -> Terminator/1
  In2/1 -> Terminator1/1
  In3/1 -> Terminator2/1
  In4/1 -> Terminator3/1
  Zero/1 -> Out1/1  "f"
  Zero1/1 -> Out2/1  "tau"
  r_sp/1 -> Terminator4/1
  theta_sp/1 -> Terminator5/1
  r_dot_sp/1 -> Terminator6/1  "r_dot_sp"
  theta_dot_sp/1 -> Terminator7/1  "theta_dot_sp"

== system robot_model/setpoint source // trajectory generator/diamond pattern 13 seconds ==
  Repeating Sequence : simulink/Sources/Repeating Sequence  rep_seq_t=[0 1 2 3 4 5 6 7 8 9 10 11 12 13]  rep_seq_y=[0 0 1 1 0 0 -1 -1 0 0 1 1 0 0]
  Repeating Sequence1 : simulink/Sources/Repeating Sequence  rep_seq_t=[0 1 2 3 4 5 6 7 8 9 10 11 12 13]  rep_seq_y=[0 0 0 0 1 1 0 0 -1 -1 0 0 0 0]
  r_sp : Outport
  theta_sp : Outport  Port=2
  wires:
  Repeating Sequence/1 -> r_sp/1  "r_sp"
  Repeating Sequence1/1 -> theta_sp/1  "theta_sp"

== system robot_model/setpoint source // trajectory generator/line pattern 9 seconds ==
  Repeating Sequence2 : simulink/Sources/Repeating Sequence  rep_seq_t=[0 1 2 3 4 5 6 7 8]  rep_seq_y=[0 0 1 1 0 0 -1 -1 0]
  Repeating Sequence3 : simulink/Sources/Repeating Sequence  rep_seq_t=[0 1 2 3 4 5 6 7 8]  rep_seq_y=[0 0 1 1 0 0 -1 -1 0]
  Out1 : Outport
  Out2 : Outport  Port=2
  wires:
  Repeating Sequence3/1 -> Out1/1
  Repeating Sequence2/1 -> Out2/1

== system robot_model/setpoint source // trajectory generator/star pattern 17 seconds ==
  Repeating Sequence : simulink/Sources/Repeating Sequence  rep_seq_t=[0 1 2 3 4 9 10 11 12 17]  rep_seq_y=[0 0 1 1 0 0 -1 -1 0 0]
  Repeating Sequence1 : simulink/Sources/Repeating Sequence  rep_seq_t=[0 5 6 7 8 13 14 15 16 17]  rep_seq_y=[0 0 1 1 0 0 -1 -1 0 0]
  r_sp : Outport
  theta_sp : Outport  Port=2
  wires:
  Repeating Sequence/1 -> r_sp/1  "r_sp"
  Repeating Sequence1/1 -> theta_sp/1  "theta_sp"

== matlab function robot_model/BOUNDARIES/BOUNDED_AREA_CHOICE/MATLAB Function1 ==
  data: x input; out output; x_dot input; x_min input; x_max input
function out = saturate_velocity(x, x_dot, x_min, x_max)
    if (x >= x_max && x_dot > 0) || (x <= x_min && x_dot < 0)
        out = 0;
    else
        out = x_dot;
    end
end

== matlab function robot_model/BOUNDARIES/BOUNDED_AREA_CHOICE/MATLAB Function ==
  data: x input; out output; x_dot input; x_min input; x_max input
function out = saturate_velocity(x, x_dot, x_min, x_max)
    if (x >= x_max && x_dot > 0) || (x <= x_min && x_dot < 0)
        out = 0;
    else
        out = x_dot;
    end
end
